simulink model "ENME562Lab5v1_physical"  (R2021a)
settings: Solver=ode1  StartTime=0.0  StopTime=20  FixedStep=0.001  RelTol=1e-3
undefined symbols (not defined in the file): HIL
libraries: quarc_library x9, simulink x4
settings Model: Creator=justi  LastModifiedBy=temit
settings DebuggingCC: ArithmeticOperatorsInVariantConditions=warning
settings SFSimCC: CustomCodeUndefinedFunction=UseInterfaceOnly

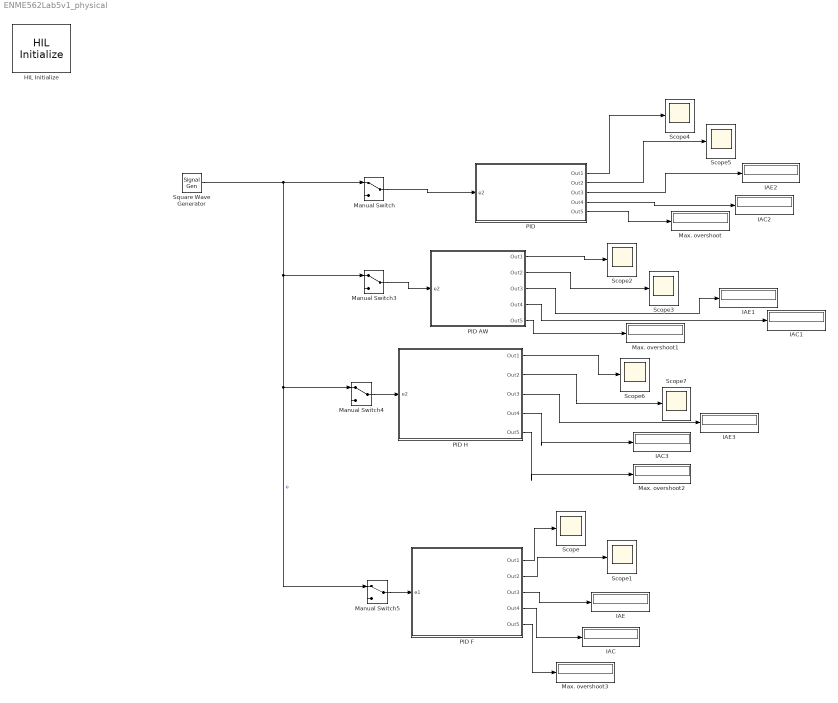
== system ENME562Lab5v1_physical ==
  HIL Initialize : quarc_library/Data Acquisition/Generic/Configuration/HIL Initialize  object_name=HIL-1  board_type=q8_usb  board_number=0  board_options=update_rate=normal;decimation=1  exclusive=off  active=on  hardware_clocks=[0:2]  clock_modes=[]  initial_clock_frequencies=[]  set_clock_params_at_start=off  set_clock_params_at_switch_in=off  set_clock_frequencies_at_start=off  set_clock_frequencies_at_switch_in=off  analog_input_channels=[0:7]  analog_input_configurations=[]  analog_input_maximums=10  analog_input_minimums=-10  set_analog_input_params_at_start=off  set_analog_input_params_at_switch_in=off  analog_output_channels=[0:7]  analog_output_maximums=10  analog_output_minimums=-10  initial_analog_outputs=[0]  final_analog_outputs=[0]  watchdog_analog_outputs=0  set_analog_output_params_at_start=off  set_analog_output_params_at_switch_in=off  set_analog_outputs_at_start=off  set_analog_outputs_at_switch_in=off  set_analog_outputs_at_terminate=off  set_analog_outputs_at_switch_out=off  set_analog_outputs_on_watchdog=off  digital_input_channels=[]  digital_output_channels=[]  digital_output_configuration=[]  initial_digital_outputs=[1]  final_digital_outputs=[1]  watchdog_digital_outputs=[1]  set_digital_output_params_at_start=off  set_digital_output_params_at_switch_in=off  set_digital_outputs_at_start=off  set_digital_outputs_at_switch_in=off  set_digital_outputs_at_terminate=off  set_digital_outputs_at_switch_out=off  set_digital_outputs_on_watchdog=off  encoder_channels=[0:7]  quadrature=[4]  encoder_filter_frequency=[]  initial_encoder_counts=[0]  set_encoder_params_at_start=off  set_encoder_params_at_switch_in=off  set_encoder_counts_at_start=off  set_encoder_counts_at_switch_in=off  pwm_channels=[0:7]  pwm_modes=0  pwm_frequency=99.532799999999995e6/4095  pwm_configuration=[0]  pwm_alignment=[0]  pwm_polarity=[1]  pwm_leading_deadband=[0]  pwm_trailing_deadband=[0]  initial_pwm_outputs=[0]  final_pwm_outputs=[0]  watchdog_pwm_outputs=[0]  set_pwm_params_at_start=off  set_pwm_params_at_switch_in=off  set_pwm_outputs_at_start=off  set_pwm_outputs_at_switch_in=off  set_pwm_outputs_at_terminate=off  set_pwm_outputs_at_switch_out=off  set_pwm_outputs_on_watchdog=off  other_output_channels=[]  initial_other_outputs=[]  final_other_outputs=[]  watchdog_other_outputs=[]  set_other_outputs_at_start=off  set_other_outputs_at_switch_in=off  set_other_outputs_at_terminate=off  set_other_outputs_at_switch_out=off  set_other_outputs_on_watchdog=off
  IAC{,1..3} (4 alike) : Display
  IAE{,1..3} (4 alike) : Display
  Manual Switch{,3..5} (4 alike) : ManualSwitch
  Max. overshoot{,1..3} (4 alike) : Display
  PID : Subsystem
  PID AW : Subsystem
  PID F : Subsystem
  PID H : Subsystem
  Scope{,1..7} (8 alike) : Scope
  Square Wave Generator : SignalGenerator  WaveForm=square  Amplitude=3  Frequency=0.2
  wires:
  PID AW/5(Out5) -> Max. overshoot1/1
  PID H/1(Out1) -> Scope6/1
  PID F/5(Out5) -> Max. overshoot3/1
  PID AW/4(Out4) -> IAC1/1
  PID F/3(Out3) -> IAE/1
  PID/5(Out5) -> Max. overshoot/1
  PID H/3(Out3) -> IAE3/1
  PID AW/2(Out2) -> Scope3/1
  PID AW/3(Out3) -> IAE1/1
  PID H/5(Out5) -> Max. overshoot2/1
  PID H/2(Out2) -> Scope7/1
  PID H/4(Out4) -> IAC3/1
  Square Wave Generator/1 -> Manual Switch3/1, Manual Switch5/1, Manual Switch4/1, Manual Switch/1  "e"
  PID/2(Out2) -> Scope5/1
  PID/1(Out1) -> Scope4/1
  PID AW/1(Out1) -> Scope2/1
  PID F/2(Out2) -> Scope1/1
  PID/3(Out3) -> IAE2/1
  Manual Switch4/1 -> PID H/1(e2)
  Manual Switch3/1 -> PID AW/1(e2)
  PID F/1(Out1) -> Scope/1
  PID F/4(Out4) -> IAC/1
  Manual Switch5/1 -> PID F/1(e1)
  PID/4(Out4) -> IAC2/1
  Manual Switch/1 -> PID/1(e2)

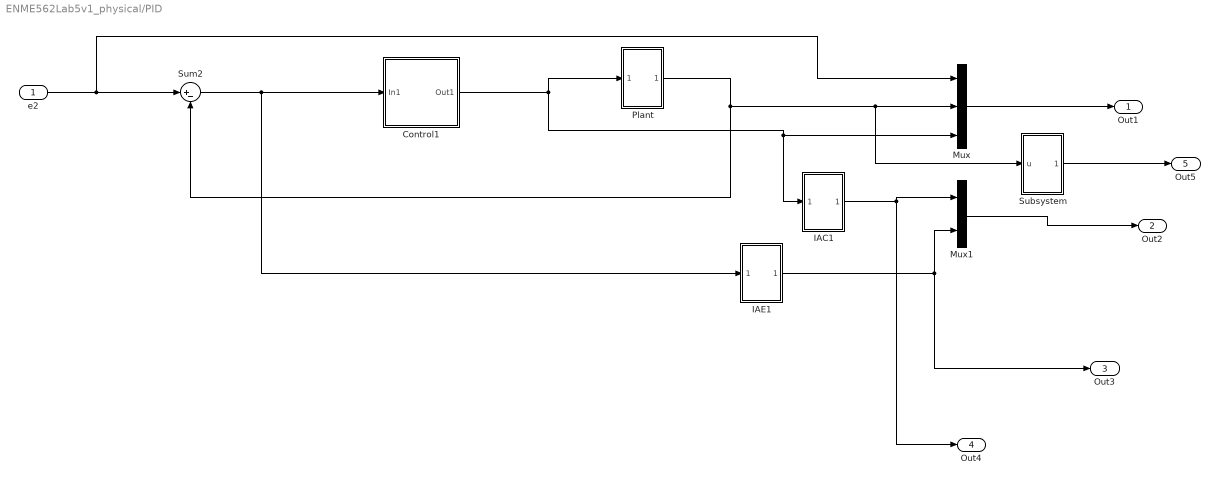
== system ENME562Lab5v1_physical/PID ==
  e2 : Inport
  Control1 : Subsystem
  IAC1 : Subsystem
  IAE1 : Subsystem
  Mux : Mux  Inputs=3
  Mux1 : Mux  Inputs=2
  Plant : Subsystem
  Subsystem : Subsystem
  Sum2 : Sum  Inputs=|+-
  Out1 : Outport
  Out2 : Outport  Port=2
  Out3 : Outport  Port=3
  Out4 : Outport  Port=4
  Out5 : Outport  Port=5
  wires:
  Mux/1 -> Out1/1
  Mux1/1 -> Out2/1
  Sum2/1 -> Control1/1(In1), IAE1/1(In1)
  IAE1/1(Out1) -> Out3/1, Mux1/2
  IAC1/1(Out1) -> Out4/1, Mux1/1
  e2/1 -> Mux/1, Sum2/1
  Control1/1(Out1) -> Plant/1(In1), Mux/3, IAC1/1(In1)
  Subsystem/1(Out1) -> Out5/1
  Plant/1(Out1) -> Sum2/2, Subsystem/1(u), Mux/2

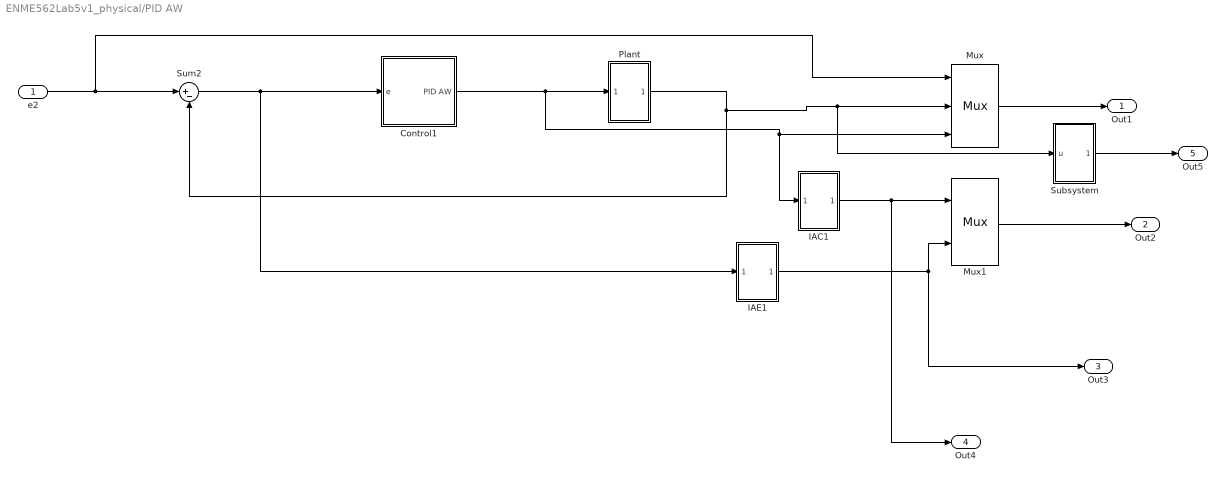
== system ENME562Lab5v1_physical/PID AW ==
  e2 : Inport
  Control1 : Subsystem
  IAC1 : Subsystem
  IAE1 : Subsystem
  Mux : Mux  Inputs=3
  Mux1 : Mux  Inputs=2
  Plant : Subsystem
  Subsystem : Subsystem
  Sum2 : Sum  Inputs=|+-
  Out1 : Outport
  Out2 : Outport  Port=2
  Out3 : Outport  Port=3
  Out4 : Outport  Port=4
  Out5 : Outport  Port=5
  wires:
  Sum2/1 -> Control1/1(e), IAE1/1(In1)
  IAC1/1(Out1) -> Out4/1, Mux1/1
  IAE1/1(Out1) -> Out3/1, Mux1/2
  e2/1 -> Mux/1, Sum2/1
  Control1/1(PID AW) -> Plant/1(In1), Mux/3, IAC1/1(In1)
  Mux1/1 -> Out2/1
  Mux/1 -> Out1/1
  Subsystem/1(Out1) -> Out5/1
  Plant/1(Out1) -> Subsystem/1(u), Mux/2, Sum2/2

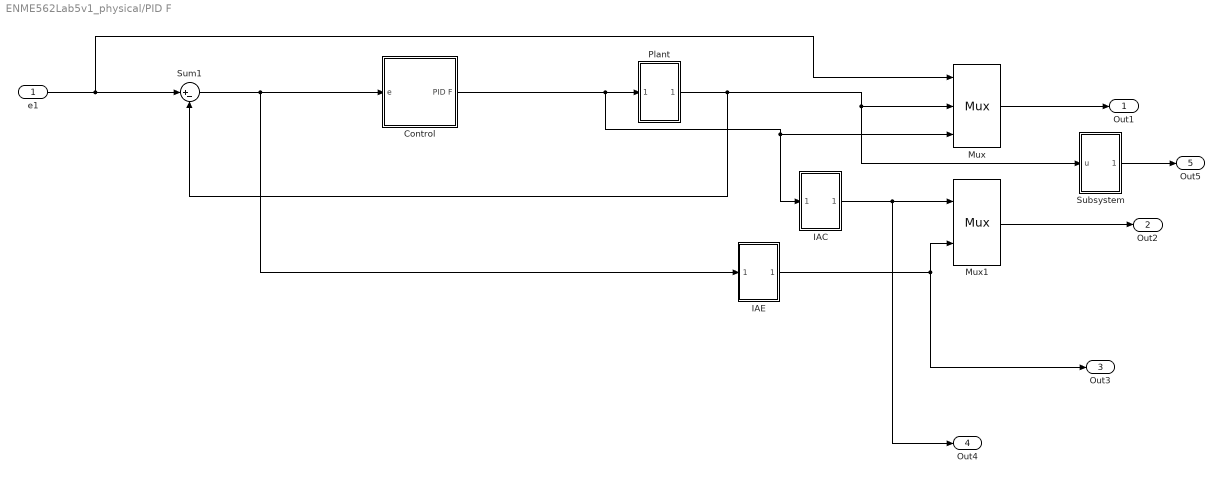
== system ENME562Lab5v1_physical/PID F ==
  e1 : Inport
  Control : Subsystem
  IAC : Subsystem
  IAE : Subsystem
  Mux : Mux  Inputs=3
  Mux1 : Mux  Inputs=2
  Plant : Subsystem
  Subsystem : Subsystem
  Sum1 : Sum  Inputs=|+-
  Out1 : Outport
  Out2 : Outport  Port=2
  Out3 : Outport  Port=3
  Out4 : Outport  Port=4
  Out5 : Outport  Port=5
  wires:
  Control/1(PID F) -> Plant/1(In1), Mux/3, IAC/1(In1)
  e1/1 -> Mux/1, Sum1/1
  IAE/1(Out1) -> Out3/1, Mux1/2
  IAC/1(Out1) -> Out4/1, Mux1/1
  Sum1/1 -> Control/1(e), IAE/1(In1)
  Mux/1 -> Out1/1
  Mux1/1 -> Out2/1
  Subsystem/1(Out1) -> Out5/1
  Plant/1(Out1) -> Subsystem/1(u), Mux/2, Sum1/2

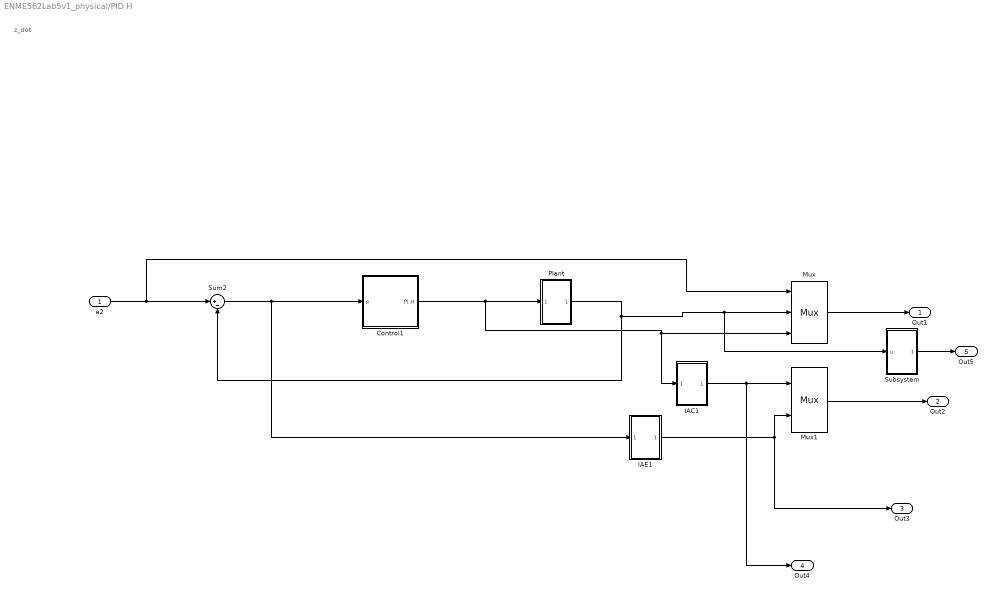
== system ENME562Lab5v1_physical/PID H ==
  note: z_dot
  e2 : Inport
  Control1 : Subsystem
  IAC1 : Subsystem
  IAE1 : Subsystem
  Mux : Mux  Inputs=3
  Mux1 : Mux  Inputs=2
  Plant : Subsystem
  Subsystem : Subsystem
  Sum2 : Sum  Inputs=|+-
  Out1 : Outport
  Out2 : Outport  Port=2
  Out3 : Outport  Port=3
  Out4 : Outport  Port=4
  Out5 : Outport  Port=5
  wires:
  Mux/1 -> Out1/1
  Mux1/1 -> Out2/1
  Sum2/1 -> Control1/1(e), IAE1/1(In1)
  IAE1/1(Out1) -> Out3/1, Mux1/2
  IAC1/1(Out1) -> Out4/1, Mux1/1
  e2/1 -> Mux/1, Sum2/1
  Control1/1(PI H) -> Plant/1(In1), Mux/3, IAC1/1(In1)
  Subsystem/1(Out1) -> Out5/1
  Plant/1(Out1) -> Subsystem/1(u), Mux/2, Sum2/2

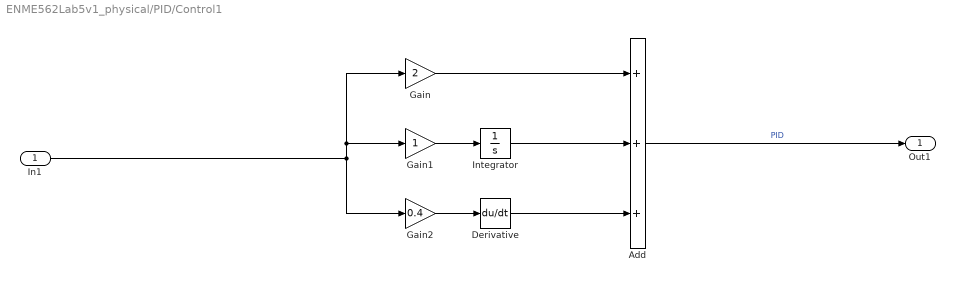
== system ENME562Lab5v1_physical/PID/Control1 ==
  In1 : Inport
  Add : Sum  Inputs=+++
  Derivative : Derivative
  Gain : Gain  Gain=2
  Gain1 : Gain
  Gain2 : Gain  Gain=0.4
  Integrator : Integrator
  Out1 : Outport
  wires:
  Gain2/1 -> Derivative/1
  Gain/1 -> Add/1
  Derivative/1 -> Add/3
  Integrator/1 -> Add/2
  Gain1/1 -> Integrator/1
  Add/1 -> Out1/1  "PID"
  In1/1 -> Gain1/1, Gain/1, Gain2/1

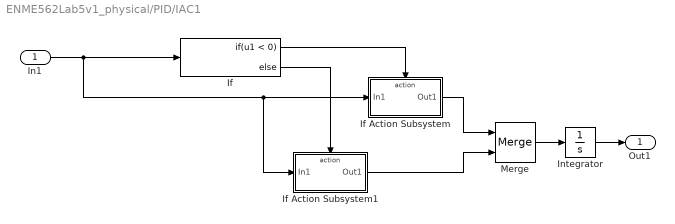
== system ENME562Lab5v1_physical/PID/IAC1 ==
  In1 : Inport
  If : If  IfExpression=u1 < 0
  If Action Subsystem : Subsystem  TreatAsAtomicUnit=on
  If Action Subsystem1 : Subsystem  TreatAsAtomicUnit=on
  Integrator : Integrator
  Merge : Merge
  Out1 : Outport
  wires:
  If/1 -> If Action Subsystem/Action
  If/2 -> If Action Subsystem1/Action
  In1/1 -> If Action Subsystem1/1(In1), If Action Subsystem/1(In1), If/1
  If Action Subsystem1/1(Out1) -> Merge/2
  Merge/1 -> Integrator/1
  If Action Subsystem/1(Out1) -> Merge/1
  Integrator/1 -> Out1/1

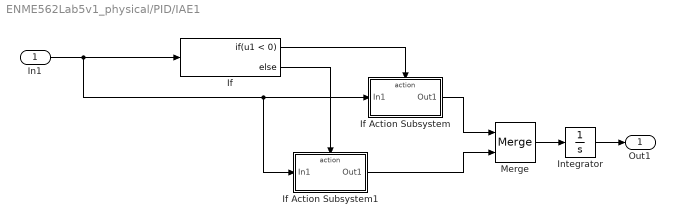
== system ENME562Lab5v1_physical/PID/IAE1 ==
  In1 : Inport
  If : If  IfExpression=u1 < 0
  If Action Subsystem : Subsystem  TreatAsAtomicUnit=on
  If Action Subsystem1 : Subsystem  TreatAsAtomicUnit=on
  Integrator : Integrator
  Merge : Merge
  Out1 : Outport
  wires:
  Integrator/1 -> Out1/1
  If Action Subsystem/1(Out1) -> Merge/1
  Merge/1 -> Integrator/1
  If Action Subsystem1/1(Out1) -> Merge/2
  In1/1 -> If/1, If Action Subsystem/1(In1), If Action Subsystem1/1(In1)
  If/2 -> If Action Subsystem1/Action
  If/1 -> If Action Subsystem/Action

== system ENME562Lab5v1_physical/PID/Plant ==
  In1 : Inport
  HIL Read Analog : quarc_library/Data Acquisition/Generic/Immediate I//O/HIL Read Analog  object_name=HIL-1  channels=0  sample_time=qc_get_step_size  active=on  vector_output=off
  HIL Write Analog : quarc_library/Data Acquisition/Generic/Immediate I//O/HIL Write Analog  object_name=HIL-1  channels=0  sample_time=-1  active=off  vector_input=off
  Out1 : Outport
  wires:
  In1/1 -> HIL Write Analog/1
  HIL Read Analog/1 -> Out1/1

== system ENME562Lab5v1_physical/PID/Subsystem ==
  u : Inport
  Constant : Constant  Value=3
  MinMax Running Resettable : simulink/Math Operations/MinMax Running Resettable  Function=max  vinit=0.0
  Subtract : Sum  Inputs=+-
  Out1 : Outport
  wires:
  Constant/1 -> Subtract/2
  MinMax Running Resettable/1 -> Subtract/1
  Subtract/1 -> Out1/1
  u/1 -> MinMax Running Resettable/1

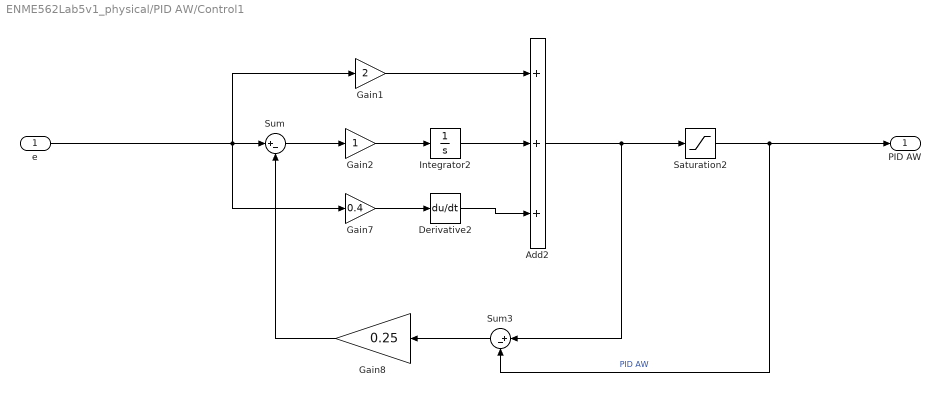
== system ENME562Lab5v1_physical/PID AW/Control1 ==
  e : Inport
  Add2 : Sum  Inputs=+++
  Derivative2 : Derivative
  Gain1 : Gain  Gain=2
  Gain2 : Gain
  Gain7 : Gain  Gain=0.4
  Gain8 : Gain  Gain=0.25
  Integrator2 : Integrator
  Saturation2 : Saturate  UpperLimit=10  LowerLimit=-10
  Sum : Sum  Inputs=|+-
  Sum3 : Sum  Inputs=|+-
  PID AW : Outport  VectorParamsAs1DForOutWhenUnconnected=off
  wires:
  e/1 -> Sum/1, Gain1/1, Gain7/1
  Sum/1 -> Gain2/1
  Integrator2/1 -> Add2/2
  Gain7/1 -> Derivative2/1
  Saturation2/1 -> PID AW/1, Sum3/2  "PID AW"
  Gain2/1 -> Integrator2/1
  Derivative2/1 -> Add2/3
  Gain1/1 -> Add2/1
  Add2/1 -> Sum3/1, Saturation2/1
  Gain8/1 -> Sum/2
  Sum3/1 -> Gain8/1

== system ENME562Lab5v1_physical/PID AW/IAC1 ==
  In1 : Inport
  If : If  IfExpression=u1 < 0
  If Action Subsystem : Subsystem  TreatAsAtomicUnit=on
  If Action Subsystem1 : Subsystem  TreatAsAtomicUnit=on
  Integrator : Integrator
  Merge : Merge
  Out1 : Outport
  wires:
  If/1 -> If Action Subsystem/Action
  If/2 -> If Action Subsystem1/Action
  In1/1 -> If Action Subsystem1/1(In1), If Action Subsystem/1(In1), If/1
  If Action Subsystem1/1(Out1) -> Merge/2
  Merge/1 -> Integrator/1
  If Action Subsystem/1(Out1) -> Merge/1
  Integrator/1 -> Out1/1

== system ENME562Lab5v1_physical/PID AW/IAE1 ==
  In1 : Inport
  If : If  IfExpression=u1 < 0
  If Action Subsystem : Subsystem  TreatAsAtomicUnit=on
  If Action Subsystem1 : Subsystem  TreatAsAtomicUnit=on
  Integrator : Integrator
  Merge : Merge
  Out1 : Outport
  wires:
  Integrator/1 -> Out1/1
  If Action Subsystem/1(Out1) -> Merge/1
  Merge/1 -> Integrator/1
  If Action Subsystem1/1(Out1) -> Merge/2
  In1/1 -> If/1, If Action Subsystem/1(In1), If Action Subsystem1/1(In1)
  If/2 -> If Action Subsystem1/Action
  If/1 -> If Action Subsystem/Action

== system ENME562Lab5v1_physical/PID AW/Plant ==
  In1 : Inport
  HIL Read Analog : quarc_library/Data Acquisition/Generic/Immediate I//O/HIL Read Analog  object_name=HIL-1  channels=0  sample_time=qc_get_step_size  active=on  vector_output=off
  HIL Write Analog : quarc_library/Data Acquisition/Generic/Immediate I//O/HIL Write Analog  object_name=HIL-1  channels=0  sample_time=-1  active=off  vector_input=off
  Out1 : Outport
  wires:
  In1/1 -> HIL Write Analog/1
  HIL Read Analog/1 -> Out1/1

== system ENME562Lab5v1_physical/PID AW/Subsystem ==
  u : Inport
  Constant : Constant  Value=3
  MinMax Running Resettable : simulink/Math Operations/MinMax Running Resettable  Function=max  vinit=0.0
  Subtract : Sum  Inputs=+-
  Out1 : Outport
  wires:
  Constant/1 -> Subtract/2
  MinMax Running Resettable/1 -> Subtract/1
  Subtract/1 -> Out1/1
  u/1 -> MinMax Running Resettable/1

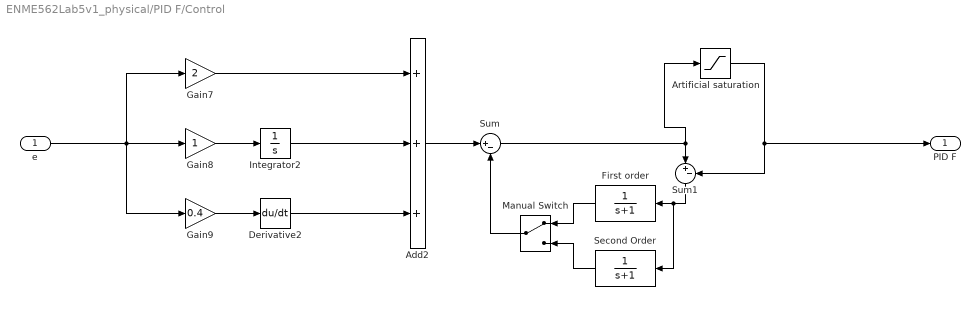
== system ENME562Lab5v1_physical/PID F/Control ==
  e : Inport
  Add2 : Sum  Inputs=+++
  Artificial saturation : Saturate  UpperLimit=10  LowerLimit=-10
  Derivative2 : Derivative
  First order : TransferFcn  Denominator=[1 1]
  Gain7 : Gain  Gain=2
  Gain8 : Gain
  Gain9 : Gain  Gain=0.4
  Integrator2 : Integrator
  Manual Switch : ManualSwitch
  Second Order : TransferFcn  Denominator=[1 1]
  Sum : Sum  Inputs=|+-
  Sum1 : Sum  Inputs=|+-
  PID F : Outport  VectorParamsAs1DForOutWhenUnconnected=off
  wires:
  e/1 -> Gain9/1, Gain8/1, Gain7/1
  Gain7/1 -> Add2/1
  Integrator2/1 -> Add2/2
  Gain8/1 -> Integrator2/1
  Derivative2/1 -> Add2/3
  Gain9/1 -> Derivative2/1
  Artificial saturation/1 -> PID F/1, Sum1/2
  Add2/1 -> Sum/1
  Sum/1 -> Sum1/1, Artificial saturation/1
  Sum1/1 -> Second Order/1, First order/1
  First order/1 -> Manual Switch/1
  Second Order/1 -> Manual Switch/2
  Manual Switch/1 -> Sum/2

== system ENME562Lab5v1_physical/PID F/IAC ==
  In1 : Inport
  If : If  IfExpression=u1 < 0
  If Action Subsystem : Subsystem  TreatAsAtomicUnit=on
  If Action Subsystem1 : Subsystem  TreatAsAtomicUnit=on
  Integrator : Integrator
  Merge : Merge
  Out1 : Outport
  wires:
  If/1 -> If Action Subsystem/Action
  If/2 -> If Action Subsystem1/Action
  In1/1 -> If Action Subsystem1/1(In1), If Action Subsystem/1(In1), If/1
  If Action Subsystem1/1(Out1) -> Merge/2
  Merge/1 -> Integrator/1
  If Action Subsystem/1(Out1) -> Merge/1
  Integrator/1 -> Out1/1

== system ENME562Lab5v1_physical/PID F/IAE ==
  In1 : Inport
  If : If  IfExpression=u1 < 0
  If Action Subsystem : Subsystem  TreatAsAtomicUnit=on
  If Action Subsystem1 : Subsystem  TreatAsAtomicUnit=on
  Integrator : Integrator
  Merge : Merge
  Out1 : Outport
  wires:
  Integrator/1 -> Out1/1
  If Action Subsystem/1(Out1) -> Merge/1
  Merge/1 -> Integrator/1
  If Action Subsystem1/1(Out1) -> Merge/2
  In1/1 -> If/1, If Action Subsystem/1(In1), If Action Subsystem1/1(In1)
  If/2 -> If Action Subsystem1/Action
  If/1 -> If Action Subsystem/Action

== system ENME562Lab5v1_physical/PID F/Plant ==
  In1 : Inport
  HIL Read Analog : quarc_library/Data Acquisition/Generic/Immediate I//O/HIL Read Analog  object_name=HIL-1  channels=0  sample_time=qc_get_step_size  active=on  vector_output=off
  HIL Write Analog : quarc_library/Data Acquisition/Generic/Immediate I//O/HIL Write Analog  object_name=HIL-1  channels=0  sample_time=-1  active=off  vector_input=off
  Out1 : Outport
  wires:
  In1/1 -> HIL Write Analog/1
  HIL Read Analog/1 -> Out1/1

== system ENME562Lab5v1_physical/PID F/Subsystem ==
  u : Inport
  Constant : Constant  Value=3
  MinMax Running Resettable : simulink/Math Operations/MinMax Running Resettable  Function=max  vinit=0.0
  Subtract : Sum  Inputs=+-
  Out1 : Outport
  wires:
  Constant/1 -> Subtract/2
  MinMax Running Resettable/1 -> Subtract/1
  Subtract/1 -> Out1/1
  u/1 -> MinMax Running Resettable/1

== system ENME562Lab5v1_physical/PID H/Control1 ==
  note: u
  note: uc
  e : Inport
  Artificial saturation : Saturate  UpperLimit=10  LowerLimit=-10
  State-Space : StateSpace  A=-1/2  B=1/2  D=2  InitialCondition=0
  Subsystem2 : Subsystem
  unfinished : Subsystem
  PI H : Outport  VectorParamsAs1DForOutWhenUnconnected=off
  wires:
  Artificial saturation/1 -> unfinished/2(u), PI H/1
  unfinished/1(uc) -> Artificial saturation/1
  e/1 -> unfinished/1(e)

== system ENME562Lab5v1_physical/PID H/IAC1 ==
  In1 : Inport
  If : If  IfExpression=u1 < 0
  If Action Subsystem : Subsystem  TreatAsAtomicUnit=on
  If Action Subsystem1 : Subsystem  TreatAsAtomicUnit=on
  Integrator : Integrator
  Merge : Merge
  Out1 : Outport
  wires:
  If/1 -> If Action Subsystem/Action
  If/2 -> If Action Subsystem1/Action
  In1/1 -> If Action Subsystem1/1(In1), If Action Subsystem/1(In1), If/1
  If Action Subsystem1/1(Out1) -> Merge/2
  Merge/1 -> Integrator/1
  If Action Subsystem/1(Out1) -> Merge/1
  Integrator/1 -> Out1/1

== system ENME562Lab5v1_physical/PID H/IAE1 ==
  In1 : Inport
  If : If  IfExpression=u1 < 0
  If Action Subsystem : Subsystem  TreatAsAtomicUnit=on
  If Action Subsystem1 : Subsystem  TreatAsAtomicUnit=on
  Integrator : Integrator
  Merge : Merge
  Out1 : Outport
  wires:
  Integrator/1 -> Out1/1
  If Action Subsystem/1(Out1) -> Merge/1
  Merge/1 -> Integrator/1
  If Action Subsystem1/1(Out1) -> Merge/2
  In1/1 -> If/1, If Action Subsystem/1(In1), If Action Subsystem1/1(In1)
  If/2 -> If Action Subsystem1/Action
  If/1 -> If Action Subsystem/Action

== system ENME562Lab5v1_physical/PID H/Plant ==
  In1 : Inport
  HIL Read Analog : quarc_library/Data Acquisition/Generic/Immediate I//O/HIL Read Analog  object_name=HIL-1  channels=0  sample_time=qc_get_step_size  active=on  vector_output=off
  HIL Write Analog : quarc_library/Data Acquisition/Generic/Immediate I//O/HIL Write Analog  object_name=HIL-1  channels=0  sample_time=-1  active=off  vector_input=off
  Out1 : Outport
  wires:
  In1/1 -> HIL Write Analog/1
  HIL Read Analog/1 -> Out1/1

== system ENME562Lab5v1_physical/PID H/Subsystem ==
  u : Inport
  Constant : Constant  Value=3
  MinMax Running Resettable : simulink/Math Operations/MinMax Running Resettable  Function=max  vinit=0.0
  Subtract : Sum  Inputs=+-
  Out1 : Outport
  wires:
  Constant/1 -> Subtract/2
  MinMax Running Resettable/1 -> Subtract/1
  Subtract/1 -> Out1/1
  u/1 -> MinMax Running Resettable/1

== system ENME562Lab5v1_physical/PID/IAC1/If Action Subsystem ==
  In1 : Inport
  Action Port : ActionPort
  Abs : Abs
  Out1 : Outport
  wires:
  In1/1 -> Abs/1
  Abs/1 -> Out1/1

== system ENME562Lab5v1_physical/PID/IAC1/If Action Subsystem1 ==
  In1 : Inport
  Action Port : ActionPort
  Out1 : Outport
  wires:
  In1/1 -> Out1/1

== system ENME562Lab5v1_physical/PID/IAE1/If Action Subsystem ==
  In1 : Inport
  Action Port : ActionPort
  Abs : Abs
  Out1 : Outport
  wires:
  Abs/1 -> Out1/1
  In1/1 -> Abs/1

== system ENME562Lab5v1_physical/PID/IAE1/If Action Subsystem1 ==
  In1 : Inport
  Action Port : ActionPort
  Out1 : Outport
  wires:
  In1/1 -> Out1/1

== system ENME562Lab5v1_physical/PID AW/IAC1/If Action Subsystem ==
  In1 : Inport
  Action Port : ActionPort
  Abs : Abs
  Out1 : Outport
  wires:
  In1/1 -> Abs/1
  Abs/1 -> Out1/1

== system ENME562Lab5v1_physical/PID AW/IAC1/If Action Subsystem1 ==
  In1 : Inport
  Action Port : ActionPort
  Out1 : Outport
  wires:
  In1/1 -> Out1/1

== system ENME562Lab5v1_physical/PID AW/IAE1/If Action Subsystem ==
  In1 : Inport
  Action Port : ActionPort
  Abs : Abs
  Out1 : Outport
  wires:
  Abs/1 -> Out1/1
  In1/1 -> Abs/1

== system ENME562Lab5v1_physical/PID AW/IAE1/If Action Subsystem1 ==
  In1 : Inport
  Action Port : ActionPort
  Out1 : Outport
  wires:
  In1/1 -> Out1/1

== system ENME562Lab5v1_physical/PID F/IAC/If Action Subsystem ==
  In1 : Inport
  Action Port : ActionPort
  Abs : Abs
  Out1 : Outport
  wires:
  In1/1 -> Abs/1
  Abs/1 -> Out1/1

== system ENME562Lab5v1_physical/PID F/IAC/If Action Subsystem1 ==
  In1 : Inport
  Action Port : ActionPort
  Out1 : Outport
  wires:
  In1/1 -> Out1/1

== system ENME562Lab5v1_physical/PID F/IAE/If Action Subsystem ==
  In1 : Inport
  Action Port : ActionPort
  Abs : Abs
  Out1 : Outport
  wires:
  Abs/1 -> Out1/1
  In1/1 -> Abs/1

== system ENME562Lab5v1_physical/PID F/IAE/If Action Subsystem1 ==
  In1 : Inport
  Action Port : ActionPort
  Out1 : Outport
  wires:
  In1/1 -> Out1/1

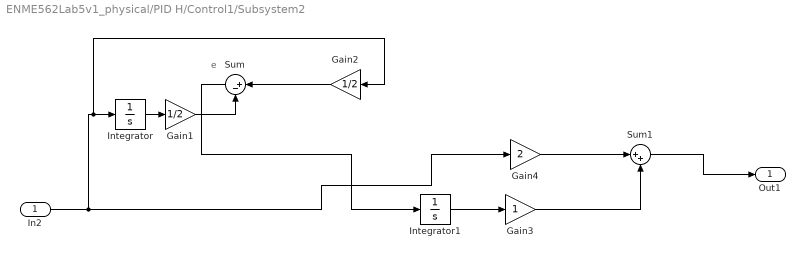
== system ENME562Lab5v1_physical/PID H/Control1/Subsystem2 ==
  note: e
  In2 : Inport
  Gain1 : Gain  Gain=1/2
  Gain2 : Gain  Gain=1/2
  Gain3 : Gain
  Gain4 : Gain  Gain=2
  Integrator : Integrator
  Integrator1 : Integrator
  Sum : Sum  Inputs=|+-
  Sum1 : Sum  Inputs=|++
  Out1 : Outport
  wires:
  Gain2/1 -> Sum/1
  Gain3/1 -> Sum1/2
  In2/1 -> Gain4/1, Gain2/1, Integrator/1
  Integrator1/1 -> Gain3/1
  Gain4/1 -> Sum1/1
  Integrator/1 -> Gain1/1
  Gain1/1 -> Sum/2
  Sum/1 -> Integrator1/1
  Sum1/1 -> Out1/1

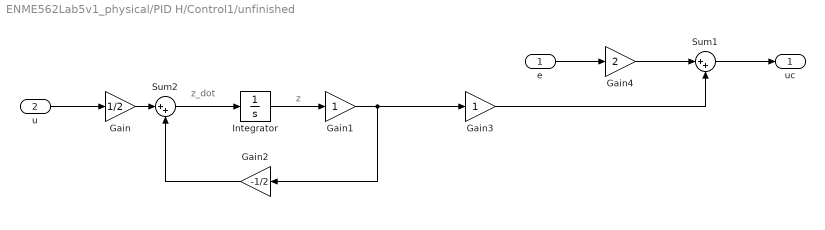
== system ENME562Lab5v1_physical/PID H/Control1/unfinished ==
  note: z_dot
  note: z
  e : Inport
  u : Inport  Port=2
  Gain : Gain  Gain=1/2
  Gain1 : Gain
  Gain2 : Gain  Gain=-1/2
  Gain3 : Gain
  Gain4 : Gain  Gain=2
  Integrator : Integrator
  Sum1 : Sum  Inputs=|++
  Sum2 : Sum  Inputs=|++
  uc : Outport
  wires:
  Gain3/1 -> Sum1/2
  e/1 -> Gain4/1
  Gain1/1 -> Gain2/1, Gain3/1
  Gain4/1 -> Sum1/1
  Integrator/1 -> Gain1/1
  Sum1/1 -> uc/1
  u/1 -> Gain/1
  Gain/1 -> Sum2/1
  Sum2/1 -> Integrator/1
  Gain2/1 -> Sum2/2

== system ENME562Lab5v1_physical/PID H/IAC1/If Action Subsystem ==
  In1 : Inport
  Action Port : ActionPort
  Abs : Abs
  Out1 : Outport
  wires:
  In1/1 -> Abs/1
  Abs/1 -> Out1/1

== system ENME562Lab5v1_physical/PID H/IAC1/If Action Subsystem1 ==
  In1 : Inport
  Action Port : ActionPort
  Out1 : Outport
  wires:
  In1/1 -> Out1/1

== system ENME562Lab5v1_physical/PID H/IAE1/If Action Subsystem ==
  In1 : Inport
  Action Port : ActionPort
  Abs : Abs
  Out1 : Outport
  wires:
  Abs/1 -> Out1/1
  In1/1 -> Abs/1

== system ENME562Lab5v1_physical/PID H/IAE1/If Action Subsystem1 ==
  In1 : Inport
  Action Port : ActionPort
  Out1 : Outport
  wires:
  In1/1 -> Out1/1
